simulink subsystem "propulsion_model"  (R2025b)
settings: Solver=VariableStepAuto  StartTime=0.0  StopTime=10.0  RelTol=1e-3
values from neighbouring files (symbols this model uses):
  a = 13.06    [params.m]    (also in params_3dof.m = 0.0013; test.m = 0.0013)
  b = 0.0859    [params.m]    (also in params_3dof.m = 8.5908; test.m = 8.5908)
  B_eff = [ ... (first row only)    [params.m]
  T_delay_actor = 20e-3    (= 0.02)    [params.m]
settings Model: Creator=schwmaxi  LastModifiedBy=schwmaxi

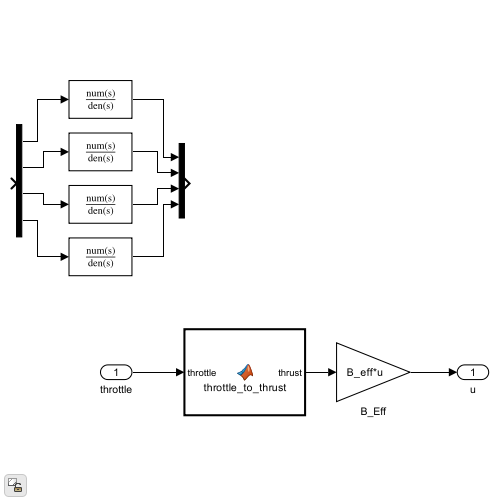
[thumbnail: Simulink's stored preview of the top-level diagram]
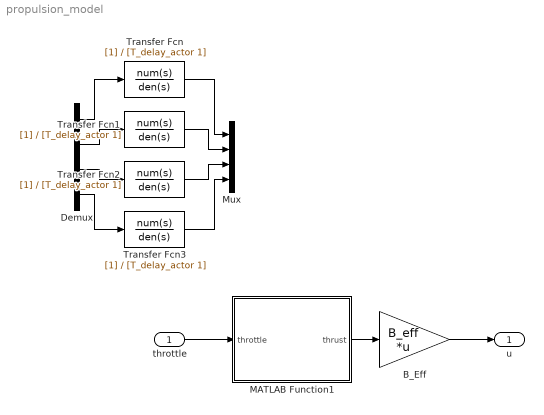
== system propulsion_model ==
  throttle : Inport
  B_Eff : Gain  Gain=B_eff  Multiplication=Matrix(K*u)
  Demux : Demux
  MATLAB Function1 : MATLAB Function  TreatAsAtomicUnit=on
  Mux : Mux
  Transfer Fcn{,1..3} (4 alike) : TransferFcn  Denominator=[T_delay_actor 1]
  u : Outport
  wires:
  B_Eff/1 -> u/1
  MATLAB Function1/1(thrust) -> B_Eff/1
  throttle/1 -> MATLAB Function1/1(throttle)
  Demux/1 -> Transfer Fcn/1
  Demux/2 -> Transfer Fcn1/1
  Transfer Fcn2/1 -> Mux/3
  Transfer Fcn/1 -> Mux/1
  Demux/3 -> Transfer Fcn2/1
  Transfer Fcn3/1 -> Mux/4
  Demux/4 -> Transfer Fcn3/1
  Transfer Fcn1/1 -> Mux/2

== matlab function propulsion_model/MATLAB Function1 ==
  data: thrust output; throttle input; a parameter; b parameter
function thrust = throttle_to_thrust(throttle, a, b)
    thrust = a * (throttle - b).^2;
end
